simulink model "Copy_of_VTOLTiltrotor"  (R2024a)
settings: configuration reference "VTOLConfiguration" (kept outside this file)
undefined symbols (not defined in the file): airspeed, Battery, BCE12, BCE_Set_init, BMS_Controller_State, C, Cell10_P, Cell11_P, Cell12_P, Cell1_N, Cell1_P, Cell2_P, Cell3_P, Cell4_P, Cell5_P, Cell6_P, Cell7_P, Cell8_P, Cell9_P, Cell_Temperatures, Cell_Voltages, Charging_State, CityMission, control, controlParams, ControlSampleTime, CriticalTiltAngle, currentFactor, CV_Gain, ddx, ddy, ddz, Device_01, DiscIntNeverNeededParam, dx, dy, dz, Earth, env, F, F28379D_ADC_MaxCount, F28379D_ADC_Vmax, FixedWingMission, flightState, Foc_Ki_IxTcpu, Foc_Ki_S, Foc_Kp_I, Foc_Kp_S, fractalcoef, FSState, FWControlParams, HoverMission, I_cc, Ia_offset, Ib_offset, iniRoll, initPitch, iniYaw, IO334, IO334_DAC_Vmax ... (+55)
libraries: slrealtimeethercatlib x109, simulink x81, fl_lib x65, slpidlib x49, mcbcontrolslib x48, nesl_utility x43, speedgoatlib_hdlCoder_IO3xx x31, canmsglib x17, slrealtimeutilitieslib x13, mcbhdlplantlib x13, speedgoatlib_IO611 x12, dspstat3 x12
(part 8 of 20)

== system Copy_of_VTOLTiltrotor/Motor Control/Three-Phase PMSM Drive/PMSM and inverter with switching dynamics/PMSM_3P2L_Inverter_Plant_TBR ==
  PCIe_RC_or_TTL : Inport
  PCIe_PWM_Config : Inport  Port=2
  PCIe_PWM_Runtime : Inport  Port=3
  PCIe_PWM_Enable : Inport  Port=4
  PCIe_Protocol : Inport  Port=5
  PCIe_V_dc : Inport  Port=6
  PCIe_Fault : Inport  Port=7
  PCIe_LdTrq/Spd : Inport  Port=8
  PCIe_Motor_Config : Inport  Port=9
  PCIe_Motor_Connection : Inport  Port=10
  PCIe_QAE_Config : Inport  Port=11
  PCIe_Resolver_Config : Inport  Port=12
  PCIe_Iabc_DAC_gain : Inport  Port=13
  PCIe_Iabc_DAC_bias : Inport  Port=14
  PCIe_DAC_reset : Inport  Port=15
  HIL_PWM_{0..5} (6 alike) : Constant  Value=0  OutDataTypeStr=boolean
  PMSM_3P2L_Inverter_Plant1 : Subsystem  mask(Speedgoat IO334-325k Interface Block){module_id=1, slot=-1, ts=-1, dacGain_1=10.0V, dacActiv_1=off, dacGain_2=2.5V, dacActiv_2=on, dacGain_3=2.5V, dacActiv_3=on, dacGain_4=2.5V, dacActiv_4=on, dacGain_5=2.5V, dacActiv_5=on, dacGain_6=10.0V, dacActiv_6=off, dacGain_7=2.5V, dacActiv_7=on, dacGain_8=10.0V, dacActiv_8=off, dacGain_9=10.0V, dacActiv_9=off, dacGain_10=10.0V, dacActiv_10=off, dacGain_11=10.0V, dacActiv_11=off, dacGain_12=10.0V, dacActiv_12=off, dacGain_13=10.0V, dacActiv_13=off, dacGain_14=10.0V, dacActiv_14=off, dacGain_15=10.0V, dacActiv_15=off, dacGain_16=10.0V, dacActiv_16=off, PullRPort0=pull-up 3.3V, VioPort0=3.3V, PullRPort1=pull-up 3.3V, VioPort1=3.3V, PullRPort2=pull-up 3.3V, VioPort2=3.3V, PullRPort3=pull-up 3.3V, VioPort3=3.3V, PullRPort4=pull-up 3.3V, VioPort4=3.3V, PullRPort5=pull-up 3.3V, VioPort5=3.3V, PullRPort6=pull-up 3.3V, VioPort6=3.3V, fpga_sync_mode=on, reset_mode=on, reset_mode_stop=on, FpgaFreq=200}
      mask prompts: module_id "FPGA Module Identifier:"; slot "PCI slot (-1: autosearch):"; ts "Sample time:"; dacGain_1 "DAC Ch 01 Range"; dacActiv_1 "Activ"; dacGain_2 "DAC Ch 02 Range"; dacActiv_2 "Activ"; dacGain_3 "DAC Ch 03 Range"; dacActiv_3 "Activ"; dacGain_4 "DAC Ch 04 Range"; dacActiv_4 "Activ"; dacGain_5 "DAC Ch 05 Range"; dacActiv_5 "Activ"; dacGain_6 "DAC Ch 06 Range"; dacActiv_6 "Activ"; dacGain_7 "DAC Ch 07 Range"; dacActiv_7 "Activ"; dacGain_8 "DAC Ch 08 Range"; dacActiv_8 "Activ"; dacGain_9 "DAC Ch 09 Range"; dacActiv_9 "Activ"; dacGain_10 "DAC Ch 10 Range"; dacActiv_10 "Activ"; dacGain_11 "DAC Ch 11 Range"; dacActiv_11 "Activ"; dacGain_12 "DAC Ch 12 Range"; dacActiv_12 "Activ"; dacGain_13 "DAC Ch 13 Range"; dacActiv_13 "Activ"; dacGain_14 "DAC Ch 14 Range"; dacActiv_14 "Activ"; dacGain_15 "DAC Ch 15 Range"; dacActiv_15 "Activ"; dacGain_16 "DAC Ch 16 Range"; dacActiv_16 "Activ"; PullRPort0 "pull resistor"; VioPort0 "I/O voltage"; PullRPort1 "pull resistor"; VioPort1 "I/O voltage"; PullRPort2 "pull resistor"; VioPort2 "I/O voltage"; PullRPort3 "pull resistor"; VioPort3 "I/O voltage"; PullRPort4 "pull resistor"; VioPort4 "I/O voltage"; PullRPort5 "pull resistor"; VioPort5 "I/O voltage"; PullRPort6 "pull resistor"; VioPort6 "I/O voltage"; fpga_sync_mode "Run FPGA only when target application runs"; reset_mode "Reset FPGA states on start"; reset_mode_stop "Reset FPGA states on stop"; FpgaFreq "FPGA Frequency [MHz]"
      mask help: Simulink Real-Time Interface Block for Speedgoat IO334-325k.
      mask init:
      | hdlslrt.backend.mfpgaparameters;
      | if sg.hdlc.utils.compareMatlabVersion('~=', 'R2023b')
      | 	sg.hdlc.warning(['The interface model that you are attempting to use was generated ',...
      | 		'in MATLAB R2023b and may not be compatible with the version you are currently using. ',...
      | 		'Attempting to use this interface model in a different MATLAB release can lead to ',...
      | 		'application crashes or other unpredictable behavior. ',...
      | 		'In order to avoid this and ensure stability and correct functionality, ',...
      | 		'we highly recommend regenerating the model with your current MATLAB release.']);
      | end
      mask Help: eval('speedgoatdoc_hdlc')
      mask TypeOptions dacGain_1: AD5547 Setup/dacGain_1
      mask TypeOptions dacActiv_1: AD5547 Setup/dacActiv_1
      mask TypeOptions dacGain_2: AD5547 Setup/dacGain_2
      mask TypeOptions dacActiv_2: AD5547 Setup/dacActiv_2
      mask TypeOptions dacGain_3: AD5547 Setup/dacGain_3
      mask TypeOptions dacActiv_3: AD5547 Setup/dacActiv_3
      mask TypeOptions dacGain_4: AD5547 Setup/dacGain_4
      mask TypeOptions dacActiv_4: AD5547 Setup/dacActiv_4
      mask TypeOptions dacGain_5: AD5547 Setup/dacGain_5
      mask TypeOptions dacActiv_5: AD5547 Setup/dacActiv_5
      mask TypeOptions dacGain_6: AD5547 Setup/dacGain_6
      mask TypeOptions dacActiv_6: AD5547 Setup/dacActiv_6
      mask TypeOptions dacGain_7: AD5547 Setup/dacGain_7
      mask TypeOptions dacActiv_7: AD5547 Setup/dacActiv_7
      mask TypeOptions dacGain_8: AD5547 Setup/dacGain_8
      mask TypeOptions dacActiv_8: AD5547 Setup/dacActiv_8
      mask TypeOptions dacGain_9: AD5547 Setup/dacGain_9
      mask TypeOptions dacActiv_9: AD5547 Setup/dacActiv_9
      mask TypeOptions dacGain_10: AD5547 Setup/dacGain_10
      mask TypeOptions dacActiv_10: AD5547 Setup/dacActiv_10
      mask TypeOptions dacGain_11: AD5547 Setup/dacGain_11
      mask TypeOptions dacActiv_11: AD5547 Setup/dacActiv_11
      mask TypeOptions dacGain_12: AD5547 Setup/dacGain_12
      mask TypeOptions dacActiv_12: AD5547 Setup/dacActiv_12
      mask TypeOptions dacGain_13: AD5547 Setup/dacGain_13
      mask TypeOptions dacActiv_13: AD5547 Setup/dacActiv_13
      mask TypeOptions dacGain_14: AD5547 Setup/dacGain_14
      mask TypeOptions dacActiv_14: AD5547 Setup/dacActiv_14
      mask TypeOptions dacGain_15: AD5547 Setup/dacGain_15
      mask TypeOptions dacActiv_15: AD5547 Setup/dacActiv_15
      mask TypeOptions dacGain_16: AD5547 Setup/dacGain_16
      mask TypeOptions dacActiv_16: AD5547 Setup/dacActiv_16
      mask TypeOptions PullRPort0: Port Settings -2x 0x00590000/PullRPort0
      mask Callback PullRPort0: sg_fpga_HDLCoder_io3xx_2x_m(2);
      mask TypeOptions VioPort0: Port Settings -2x 0x00590000/VioPort0
      mask Callback VioPort0: sg_fpga_HDLCoder_io3xx_2x_m(2);
      mask TypeOptions PullRPort1: Port Settings -2x 0x00590000/PullRPort1
      mask Callback PullRPort1: sg_fpga_HDLCoder_io3xx_2x_m(2);
      mask TypeOptions VioPort1: Port Settings -2x 0x00590000/VioPort1
      mask Callback VioPort1: sg_fpga_HDLCoder_io3xx_2x_m(2);
      mask TypeOptions PullRPort2: Port Settings -2x 0x00590000/PullRPort2
      mask Callback PullRPort2: sg_fpga_HDLCoder_io3xx_2x_m(2);
      mask TypeOptions VioPort2: Port Settings -2x 0x00590000/VioPort2
      mask Callback VioPort2: sg_fpga_HDLCoder_io3xx_2x_m(2);
      mask TypeOptions PullRPort3: Port Settings -2x 0x00590000/PullRPort3
      mask Callback PullRPort3: sg_fpga_HDLCoder_io3xx_2x_m(2);
      mask TypeOptions VioPort3: Port Settings -2x 0x00590000/VioPort3
      mask Callback VioPort3: sg_fpga_HDLCoder_io3xx_2x_m(2);
      mask TypeOptions PullRPort4: Port Settings -2x 0x00590000/PullRPort4
      mask Callback PullRPort4: sg_fpga_HDLCoder_io3xx_2x_m(2);
      mask TypeOptions VioPort4: Port Settings -2x 0x00590000/VioPort4
      mask Callback VioPort4: sg_fpga_HDLCoder_io3xx_2x_m(2);
      mask TypeOptions PullRPort5: Port Settings -2x 0x00590000/PullRPort5
      mask Callback PullRPort5: sg_fpga_HDLCoder_io3xx_2x_m(2);
      mask TypeOptions VioPort5: Port Settings -2x 0x00590000/VioPort5
      mask Callback VioPort5: sg_fpga_HDLCoder_io3xx_2x_m(2);
      mask TypeOptions PullRPort6: Port Settings -2x 0x00590000/PullRPort6
      mask Callback PullRPort6: sg_fpga_HDLCoder_io3xx_2x_m(2);
      mask TypeOptions VioPort6: Port Settings -2x 0x00590000/VioPort6
      mask Callback VioPort6: sg_fpga_HDLCoder_io3xx_2x_m(2);
      mask TypeOptions fpga_sync_mode: IO3xx Setup/fpga_sync_mode
      mask TypeOptions reset_mode: IO3xx Setup/reset_mode
      mask TypeOptions reset_mode_stop: IO3xx Setup/reset_mode_stop
      mask DialogControl DAC Prompt: DAC
      mask DialogControl dacGrp_1 Prompt: Ch 01 to 08
      mask DialogControl dacGrp_2 Prompt: Ch 09 to 16
      mask DialogControl IO33421 Prompt: IO334-21
      mask DialogControl port1 Prompt: Port 1
      mask DialogControl port2 Prompt: Port 2
      mask DialogControl port3 Prompt: Port 3
      mask DialogControl port4 Prompt: Port 4
      mask DialogControl port5 Prompt: Port 5
      mask DialogControl port6 Prompt: Port 6
      mask DialogControl port7 Prompt: Port 7
      mask Display:
      | SetupBlkPath = sghdlc.model.findSystem(gcb, 'LookUnderMasks', 'all', 'FollowLinks', 'on', 'regexp', 'on', 'Name', 'IO3(\d|x){2}\s+Setup' );
      | SetupBlkPath = SetupBlkPath{1};
      | TS = get_param(SetupBlkPath,'timestamp_mcs');
      | disp(sprintf('Speedgoat IO334-325k\nFPGA I/O Module\n\nTimestamp\n%s\n\nReference Design\nVersion 1.0\n\nMATLAB R2023b\n\nPCIe Link Width: X4\nTiming Severity: error\nRear Plugin: -21\nAurora Mode: None\nAurora Crc: true\nAurora Byteswap: true\nVerifier: off\nVerifier: JTAG\n', TS))
  Terminator{,1..10} (11 alike) : Terminator
  PCIe_Ia : Outport
  PCIe_Ib : Outport  Port=2
  PCIe_Ic : Outport  Port=3
  PCIe_Idc : Outport  Port=4
  PCIe_Motor_Spd : Outport  Port=5
  PCIe_Motor_Angle : Outport  Port=6
  PCIe_Motor_ElecAngle : Outport  Port=7
  PCIe_Motor_Trq : Outport  Port=8
  PCIe_Rsvl_excitation_pos : Outport  Port=9
  PCIe_Rsvl_excitation_neg : Outport  Port=10
  PCIe_Rsvl_sin_neg : Outport  Port=11
  PCIe_Rsvl_cos_neg : Outport  Port=12
  PCIe_Resolver_Out : Outport  Port=13
  wires:
  PCIe_RC_or_TTL/1 -> PMSM_3P2L_Inverter_Plant1/1(PCIe_RC_or_TTL)
  PCIe_PWM_Config/1 -> PMSM_3P2L_Inverter_Plant1/2(PCIe_PWM_Config)
  PCIe_PWM_Runtime/1 -> PMSM_3P2L_Inverter_Plant1/3(PCIe_PWM_Runtime)
  PCIe_PWM_Enable/1 -> PMSM_3P2L_Inverter_Plant1/4(PCIe_PWM_Enable)
  PCIe_Protocol/1 -> PMSM_3P2L_Inverter_Plant1/5(PCIe_Protocol)
  PCIe_V_dc/1 -> PMSM_3P2L_Inverter_Plant1/12(PCIe_V_dc)
  PCIe_Fault/1 -> PMSM_3P2L_Inverter_Plant1/13(PCIe_Fault)
  PCIe_LdTrq/Spd/1 -> PMSM_3P2L_Inverter_Plant1/14(PCIe_LdTrq/Spd)
  PCIe_Motor_Config/1 -> PMSM_3P2L_Inverter_Plant1/15(PCIe_Motor_Config)
  PCIe_Motor_Connection/1 -> PMSM_3P2L_Inverter_Plant1/16(PCIe_Motor_Connection)
  PCIe_QAE_Config/1 -> PMSM_3P2L_Inverter_Plant1/17(PCIe_QAE_Config)
  PCIe_Resolver_Config/1 -> PMSM_3P2L_Inverter_Plant1/18(PCIe_Resolver_Config)
  PCIe_DAC_reset/1 -> PMSM_3P2L_Inverter_Plant1/21(PCIe_DAC_reset)
  PCIe_Iabc_DAC_bias/1 -> PMSM_3P2L_Inverter_Plant1/20(PCIe_Iabc_DAC_bias)
  PCIe_Iabc_DAC_gain/1 -> PMSM_3P2L_Inverter_Plant1/19(PCIe_Iabc_DAC_gain)
  PMSM_3P2L_Inverter_Plant1/1(PCIe_Ia) -> PCIe_Ia/1
  PMSM_3P2L_Inverter_Plant1/3(PCIe_Ic) -> PCIe_Ic/1
  PMSM_3P2L_Inverter_Plant1/2(PCIe_Ib) -> PCIe_Ib/1
  PMSM_3P2L_Inverter_Plant1/7(PCIe_Idc) -> PCIe_Idc/1
  PMSM_3P2L_Inverter_Plant1/8(PCIe_Motor_Spd) -> PCIe_Motor_Spd/1
  PMSM_3P2L_Inverter_Plant1/9(PCIe_Motor_Angle) -> PCIe_Motor_Angle/1
  PMSM_3P2L_Inverter_Plant1/10(PCIe_Motor_ElecAngle) -> PCIe_Motor_ElecAngle/1
  PMSM_3P2L_Inverter_Plant1/11(PCIe_Motor_Trq) -> PCIe_Motor_Trq/1
  PMSM_3P2L_Inverter_Plant1/15(PCIe_Rsvl_excitation_pos) -> PCIe_Rsvl_excitation_pos/1
  PMSM_3P2L_Inverter_Plant1/16(PCIe_Rsvl_excitation_neg) -> PCIe_Rsvl_excitation_neg/1
  PMSM_3P2L_Inverter_Plant1/17(AO_5_Rsvl_sin_pos) -> Terminator10/1  "F28379D_A5"
  PMSM_3P2L_Inverter_Plant1/18(PCIe_Rsvl_sin_neg) -> PCIe_Rsvl_sin_neg/1
  PMSM_3P2L_Inverter_Plant1/20(PCIe_Rsvl_cos_neg) -> PCIe_Rsvl_cos_neg/1
  PMSM_3P2L_Inverter_Plant1/21(PCIe_Resolver_Out) -> PCIe_Resolver_Out/1
  PMSM_3P2L_Inverter_Plant1/22(TTL_32_Protocol) -> Terminator/1  "GPIO40"
  PMSM_3P2L_Inverter_Plant1/23(TTL_24_AO_trigger_1_8) -> Terminator1/1
  PMSM_3P2L_Inverter_Plant1/24(1_8_Null_AO_trigger) -> Terminator2/1
  PMSM_3P2L_Inverter_Plant1/19(AO_7_Rsvl_cos_pos) -> Terminator3/1  "F28379D_C5"
  PMSM_3P2L_Inverter_Plant1/14("TTL_50_QEP_A_I   ") -> Terminator6/1
  PMSM_3P2L_Inverter_Plant1/12(TTL_48_QEP_A_A) -> Terminator4/1
  PMSM_3P2L_Inverter_Plant1/13(TTL_49_QEP_A_B) -> Terminator5/1
  PMSM_3P2L_Inverter_Plant1/6(AO_4_Ic) -> Terminator9/1  "F28379D_C4"
  PMSM_3P2L_Inverter_Plant1/4(AO_2_Ia) -> Terminator7/1  "F28379D_A4"
  PMSM_3P2L_Inverter_Plant1/5(AO_3_Ib) -> Terminator8/1  "F28379D_B4"
  HIL_PWM_0/1 -> PMSM_3P2L_Inverter_Plant1/6(PWM1A TTL_0)
  HIL_PWM_1/1 -> PMSM_3P2L_Inverter_Plant1/7(PWM1B TTL_1)
  HIL_PWM_2/1 -> PMSM_3P2L_Inverter_Plant1/8(PWM2A TTL_2)
  HIL_PWM_3/1 -> PMSM_3P2L_Inverter_Plant1/9(PWM2B TTL_3)
  HIL_PWM_4/1 -> PMSM_3P2L_Inverter_Plant1/10(PWM3A TTL_4)
  HIL_PWM_5/1 -> PMSM_3P2L_Inverter_Plant1/11(PWM3B TTL_5)

== system Copy_of_VTOLTiltrotor/Motor Control/Three-Phase PMSM Drive1/PMSM and average inverter/Encoder Simulation ==
  Theta_m : Inport
  Add1 : Sum  RndMeth=Simplest
  Data Type Conversion7 : DataTypeConversion  OutDataTypeStr=uint16  RndMeth=Simplest  SaturateOnIntegerOverflow=off
  "Get_PU " : Subsystem
  IndexOffset in PU : Constant  Value=0  OutDataTypeStr=single  SampleTime=-1
  Wrap : Subsystem
  pmsm.QEPSlits*4 : Gain  Gain=Maxon_Mile_Nslits*4  OutDataTypeStr=uint16  RndMeth=Simplest
  QEP_Position_Count : Outport
  wires:
  Add1/1 -> Wrap/1(in)
  Theta_m/1 -> "Get_PU "/1(rad)
  pmsm.QEPSlits*4/1 -> Data Type Conversion7/1  "Theta_e"
  Wrap/1(out) -> pmsm.QEPSlits*4/1  "theta_m(ideal)"
  IndexOffset in PU/1 -> Add1/2
  "Get_PU "/1(PU) -> Add1/1
  Data Type Conversion7/1 -> QEP_Position_Count/1

== system Copy_of_VTOLTiltrotor/Motor Control/Three-Phase PMSM Drive1/PMSM and average inverter/Ideal Inverter ==
  V_DC : Inport
  Duty Cycle abc : Inport  Port=2
  Data Type Conversion : DataTypeConversion  OutDataTypeStr=single  SaturateOnIntegerOverflow=off  RndMeth=Floor
  Demux : Demux  Outputs=3
  Mux : Mux  Inputs=3
  Product : Product
  Product1 : Product
  Product2 : Product
  Vabc : Outport
  wires:
  V_DC/1 -> Product2/1, Product1/1, Product/1
  Demux/1 -> Product/2
  Duty Cycle abc/1 -> Data Type Conversion/1
  Mux/1 -> Vabc/1
  Data Type Conversion/1 -> Demux/1
  Demux/2 -> Product1/2
  Demux/3 -> Product2/2
  Product/1 -> Mux/1
  Product1/1 -> Mux/2
  Product2/1 -> Mux/3

== system Copy_of_VTOLTiltrotor/Motor Control/Three-Phase PMSM Drive1/PMSM and average inverter/PMSM ==
  Config : Inport
  PhaseVolt abc : Inport  Port=2
  LdTrq / Spd : Inport  Port=3
  Constant : Constant  Value=0  OutDataTypeStr=boolean
  PMSM HDL : mcbhdlplantlib/PMSM HDL  VariantControl=pmsmVariant==pmsmEnum.TorqueInput  Ts=-1
      settings: LibrarySourceBlock=mcbhdllib/Electrical Systems/Motors/PMSM HDL
  Info : Outport
  PhaseCurr : Outport  Port=2
  Torque : Outport  Port=3
  RotorMechSpd : Outport  Port=4
  RotorElecAngle : Outport  Port=5
  wires:
  PMSM HDL/5 -> RotorElecAngle/1
  Config/1 -> PMSM HDL/1
  PMSM HDL/4 -> RotorMechSpd/1
  PMSM HDL/3 -> Torque/1
  PMSM HDL/2 -> PhaseCurr/1
  LdTrq / Spd/1 -> PMSM HDL/3
  PhaseVolt abc/1 -> PMSM HDL/2
  PMSM HDL/1 -> Info/1
  Constant/1 -> PMSM HDL/4

== system Copy_of_VTOLTiltrotor/Motor Control/Three-Phase PMSM Drive1/PMSM and average inverter/Runtime to DC ==
  PWM_Runtime : Inport
  Demux : Demux  Outputs=15
  Mux : Mux  Inputs=3
  To Dc A1 : Subsystem
  To Dc A2 : Subsystem
  To Dc A3 : Subsystem
  Duty Cycle abc : Outport
  wires:
  PWM_Runtime/1 -> Demux/1  "PCIe_PWM_Runtime"
  Demux/2 -> To Dc A1/1(A_on)
  Demux/3 -> To Dc A1/2(A_off)
  Demux/7 -> To Dc A2/1(A_on)
  Demux/8 -> To Dc A2/2(A_off)
  Demux/12 -> To Dc A3/1(A_on)
  Demux/13 -> To Dc A3/2(A_off)
  To Dc A1/1(Dc) -> Mux/1
  To Dc A2/1(Dc) -> Mux/2
  To Dc A3/1(Dc) -> Mux/3
  Mux/1 -> Duty Cycle abc/1

== system Copy_of_VTOLTiltrotor/Motor Control/Three-Phase PMSM Drive2/PMSM and average inverter/Encoder Simulation ==
  Theta_m : Inport
  Add1 : Sum  RndMeth=Simplest
  Data Type Conversion7 : DataTypeConversion  OutDataTypeStr=uint16  RndMeth=Simplest  SaturateOnIntegerOverflow=off
  "Get_PU " : Subsystem
  IndexOffset in PU : Constant  Value=0  OutDataTypeStr=single  SampleTime=-1
  Wrap : Subsystem
  pmsm.QEPSlits*4 : Gain  Gain=Maxon_Mile_Nslits*4  OutDataTypeStr=uint16  RndMeth=Simplest
  QEP_Position_Count : Outport
  wires:
  Add1/1 -> Wrap/1(in)
  Theta_m/1 -> "Get_PU "/1(rad)
  pmsm.QEPSlits*4/1 -> Data Type Conversion7/1  "Theta_e"
  Wrap/1(out) -> pmsm.QEPSlits*4/1  "theta_m(ideal)"
  IndexOffset in PU/1 -> Add1/2
  "Get_PU "/1(PU) -> Add1/1
  Data Type Conversion7/1 -> QEP_Position_Count/1

== system Copy_of_VTOLTiltrotor/Motor Control/Three-Phase PMSM Drive2/PMSM and average inverter/Ideal Inverter ==
  V_DC : Inport
  Duty Cycle abc : Inport  Port=2
  Data Type Conversion : DataTypeConversion  OutDataTypeStr=single  SaturateOnIntegerOverflow=off  RndMeth=Floor
  Demux : Demux  Outputs=3
  Mux : Mux  Inputs=3
  Product : Product
  Product1 : Product
  Product2 : Product
  Vabc : Outport
  wires:
  V_DC/1 -> Product2/1, Product1/1, Product/1
  Demux/1 -> Product/2
  Duty Cycle abc/1 -> Data Type Conversion/1
  Mux/1 -> Vabc/1
  Data Type Conversion/1 -> Demux/1
  Demux/2 -> Product1/2
  Demux/3 -> Product2/2
  Product/1 -> Mux/1
  Product1/1 -> Mux/2
  Product2/1 -> Mux/3

== system Copy_of_VTOLTiltrotor/Motor Control/Three-Phase PMSM Drive2/PMSM and average inverter/PMSM ==
  Config : Inport
  PhaseVolt abc : Inport  Port=2
  LdTrq / Spd : Inport  Port=3
  Constant : Constant  Value=0  OutDataTypeStr=boolean
  PMSM HDL : mcbhdlplantlib/PMSM HDL  VariantControl=pmsmVariant==pmsmEnum.TorqueInput  Ts=-1
      settings: LibrarySourceBlock=mcbhdllib/Electrical Systems/Motors/PMSM HDL
  Info : Outport
  PhaseCurr : Outport  Port=2
  Torque : Outport  Port=3
  RotorMechSpd : Outport  Port=4
  RotorElecAngle : Outport  Port=5
  wires:
  PMSM HDL/5 -> RotorElecAngle/1
  Config/1 -> PMSM HDL/1
  PMSM HDL/4 -> RotorMechSpd/1
  PMSM HDL/3 -> Torque/1
  PMSM HDL/2 -> PhaseCurr/1
  LdTrq / Spd/1 -> PMSM HDL/3
  PhaseVolt abc/1 -> PMSM HDL/2
  PMSM HDL/1 -> Info/1
  Constant/1 -> PMSM HDL/4

== system Copy_of_VTOLTiltrotor/Motor Control/Three-Phase PMSM Drive2/PMSM and average inverter/Runtime to DC ==
  PWM_Runtime : Inport
  Demux : Demux  Outputs=15
  Mux : Mux  Inputs=3
  To Dc A1 : Subsystem
  To Dc A2 : Subsystem
  To Dc A3 : Subsystem
  Duty Cycle abc : Outport
  wires:
  PWM_Runtime/1 -> Demux/1  "PCIe_PWM_Runtime"
  Demux/2 -> To Dc A1/1(A_on)
  Demux/3 -> To Dc A1/2(A_off)
  Demux/7 -> To Dc A2/1(A_on)
  Demux/8 -> To Dc A2/2(A_off)
  Demux/12 -> To Dc A3/1(A_on)
  Demux/13 -> To Dc A3/2(A_off)
  To Dc A1/1(Dc) -> Mux/1
  To Dc A2/1(Dc) -> Mux/2
  To Dc A3/1(Dc) -> Mux/3
  Mux/1 -> Duty Cycle abc/1

== system Copy_of_VTOLTiltrotor/Motor Control/Three-Phase PMSM Drive3/PMSM and average inverter/Encoder Simulation ==
  Theta_m : Inport
  Add1 : Sum  RndMeth=Simplest
  Data Type Conversion7 : DataTypeConversion  OutDataTypeStr=uint16  RndMeth=Simplest  SaturateOnIntegerOverflow=off
  "Get_PU " : Subsystem
  IndexOffset in PU : Constant  Value=0  OutDataTypeStr=single  SampleTime=-1
  Wrap : Subsystem
  pmsm.QEPSlits*4 : Gain  Gain=Maxon_Mile_Nslits*4  OutDataTypeStr=uint16  RndMeth=Simplest
  QEP_Position_Count : Outport
  wires:
  Add1/1 -> Wrap/1(in)
  Theta_m/1 -> "Get_PU "/1(rad)
  pmsm.QEPSlits*4/1 -> Data Type Conversion7/1  "Theta_e"
  Wrap/1(out) -> pmsm.QEPSlits*4/1  "theta_m(ideal)"
  IndexOffset in PU/1 -> Add1/2
  "Get_PU "/1(PU) -> Add1/1
  Data Type Conversion7/1 -> QEP_Position_Count/1

== system Copy_of_VTOLTiltrotor/Motor Control/Three-Phase PMSM Drive3/PMSM and average inverter/Ideal Inverter ==
  V_DC : Inport
  Duty Cycle abc : Inport  Port=2
  Data Type Conversion : DataTypeConversion  OutDataTypeStr=single  SaturateOnIntegerOverflow=off  RndMeth=Floor
  Demux : Demux  Outputs=3
  Mux : Mux  Inputs=3
  Product : Product
  Product1 : Product
  Product2 : Product
  Vabc : Outport
  wires:
  V_DC/1 -> Product2/1, Product1/1, Product/1
  Demux/1 -> Product/2
  Duty Cycle abc/1 -> Data Type Conversion/1
  Mux/1 -> Vabc/1
  Data Type Conversion/1 -> Demux/1
  Demux/2 -> Product1/2
  Demux/3 -> Product2/2
  Product/1 -> Mux/1
  Product1/1 -> Mux/2
  Product2/1 -> Mux/3

== system Copy_of_VTOLTiltrotor/Motor Control/Three-Phase PMSM Drive3/PMSM and average inverter/PMSM ==
  Config : Inport
  PhaseVolt abc : Inport  Port=2
  LdTrq / Spd : Inport  Port=3
  Constant : Constant  Value=0  OutDataTypeStr=boolean
  PMSM HDL : mcbhdlplantlib/PMSM HDL  VariantControl=pmsmVariant==pmsmEnum.TorqueInput  Ts=-1
      settings: LibrarySourceBlock=mcbhdllib/Electrical Systems/Motors/PMSM HDL
  Info : Outport
  PhaseCurr : Outport  Port=2
  Torque : Outport  Port=3
  RotorMechSpd : Outport  Port=4
  RotorElecAngle : Outport  Port=5
  wires:
  PMSM HDL/5 -> RotorElecAngle/1
  Config/1 -> PMSM HDL/1
  PMSM HDL/4 -> RotorMechSpd/1
  PMSM HDL/3 -> Torque/1
  PMSM HDL/2 -> PhaseCurr/1
  LdTrq / Spd/1 -> PMSM HDL/3
  PhaseVolt abc/1 -> PMSM HDL/2
  PMSM HDL/1 -> Info/1
  Constant/1 -> PMSM HDL/4

== system Copy_of_VTOLTiltrotor/Motor Control/Three-Phase PMSM Drive3/PMSM and average inverter/Runtime to DC ==
  PWM_Runtime : Inport
  Demux : Demux  Outputs=15
  Mux : Mux  Inputs=3
  To Dc A1 : Subsystem
  To Dc A2 : Subsystem
  To Dc A3 : Subsystem
  Duty Cycle abc : Outport
  wires:
  PWM_Runtime/1 -> Demux/1  "PCIe_PWM_Runtime"
  Demux/2 -> To Dc A1/1(A_on)
  Demux/3 -> To Dc A1/2(A_off)
  Demux/7 -> To Dc A2/1(A_on)
  Demux/8 -> To Dc A2/2(A_off)
  Demux/12 -> To Dc A3/1(A_on)
  Demux/13 -> To Dc A3/2(A_off)
  To Dc A1/1(Dc) -> Mux/1
  To Dc A2/1(Dc) -> Mux/2
  To Dc A3/1(Dc) -> Mux/3
  Mux/1 -> Duty Cycle abc/1

== system Copy_of_VTOLTiltrotor/Battery Management System/BMS/HIL/Controller/PLANT-Rx ==
  CAN Read : speedgoatlib_IO611/Legacy/CAN/CAN Read  id=1  sampleTime=-1  portSelection=2  messageType=CAN  BusOutput=off  protl=IO611  ptIdx=1  isFDMod=1
      settings: SourceProductName=IO611
  Data Type Conversion{,1..3} (4 alike) : DataTypeConversion  OutDataTypeStr=single  SaturateOnIntegerOverflow=off  RndMeth=Floor
  Messages : Subsystem
  While Iterator : WhileIterator  MaxIters=-1  WhileBlockType=do-while
  BMS_Faults : Outport
  Charging_State : Outport  Port=2
  BMS_State : Outport  Port=3
  SOC : Outport  Port=4
  Discharge_Current_Limit : Outport  Port=5
  Charge_Current_Limit : Outport  Port=6
  Charge_Current_Req : Outport  Port=7
  wires:
  CAN Read/2 -> Messages/4(ID_0x502), Messages/3(ID_0x501), Messages/2(ID_0x202), Messages/1(ID_0x201)
  CAN Read/1 -> While Iterator/1
  Messages/1(Discharge_Current_Limit) -> Data Type Conversion/1
  Messages/7(Charging_State) -> Charging_State/1
  Messages/2(Charge_Current_Limit) -> Data Type Conversion1/1
  Messages/3(Charge_Current_Req) -> Data Type Conversion2/1
  Messages/4(SOC) -> Data Type Conversion3/1
  Messages/6(BMS_State) -> BMS_State/1
  Data Type Conversion/1 -> Discharge_Current_Limit/1
  Data Type Conversion1/1 -> Charge_Current_Limit/1
  Data Type Conversion2/1 -> Charge_Current_Req/1
  Data Type Conversion3/1 -> SOC/1
  Messages/5(BMS_Faults) -> BMS_Faults/1

== system Copy_of_VTOLTiltrotor/Battery Management System/BMS/HIL/Controller/PLANT-Tx ==
  to_Controller : Inport
  to_Controller_SRE : Inport  Port=2
  12-Cell : Subsystem  VariantControl=Ns_Module == 12
  wires:
  to_Controller/1 -> 12-Cell/1(to_Controller)
  to_Controller_SRE/1 -> 12-Cell/2(to_Controller_SRE)

== system Copy_of_VTOLTiltrotor/Battery Management System/BMS/MIL/Cell Monitoring Unit/Balancing_Circuit ==
  Bal_Cmd_Controller : Inport
  12-Cell : Subsystem  VariantControl=Ns_Module == 12
  Cells : PMIOPort  Side=Left
  Balancing_Currents : Outport
  wires:
  Bal_Cmd_Controller/1 -> 12-Cell/1(Bal_Cmd_Controller)
  12-Cell/1(Balancing_Currents) -> Balancing_Currents/1
  connections:
  Cells/RConn1 -- 12-Cell/LConn1

== system Copy_of_VTOLTiltrotor/Battery Management System/BMS/MIL/Controller/BMS State Machine ==
  Discharge_Current_Limit : Inport
  Charge_Current_Limit : Inport  Port=2
  State_Request : Inport  Port=3  OutDataTypeStr=Enum: SRE
  Sensor_Values : Inport  Port=4
  Fault_Reset_Enable : Inport  Port=5
  Bus Selector : BusSelector  OutputSignals=Cell_Voltages,Pack_Voltage,Cell_Temperatures,Pack_Current
  Data Type Conversion : DataTypeConversion  OutDataTypeStr=boolean  SaturateOnIntegerOverflow=off  RndMeth=Floor
  State_Machine : Stateflow chart  TreatAsAtomicUnit=on  VariantControl=(default)
  Charge_Current_Req : Outport  OutMin=-100  OutMax=100  OutDataTypeStr=single  VectorParamsAs1DForOutWhenUnconnected=off
  Faults : Outport  Port=2  OutDataTypeStr=Bus: Faults  VectorParamsAs1DForOutWhenUnconnected=off  BusOutputAsStruct=on
  Charging_State : Outport  Port=3
  BMS_State : Outport  Port=4  OutDataTypeStr=Enum: BMS_Controller_State  VectorParamsAs1DForOutWhenUnconnected=off
  wires:
  State_Machine/2(Fault_out) -> Faults/1  "Faults"
  Bus Selector/1 -> State_Machine/4(Cell_Voltages)  "<Cell_Voltages>"
  State_Machine/1(ChargeCurrentReq) -> Charge_Current_Req/1  "Charge_Current_Req"
  State_Request/1 -> State_Machine/3(State_Request)
  Discharge_Current_Limit/1 -> State_Machine/1(DischargeCurrentLimit)
  Charge_Current_Limit/1 -> State_Machine/2(ChargeCurrentLimit)
  Bus Selector/3 -> State_Machine/6(Cell_Temperatures)  "<Cell_Temperatures>"
  Bus Selector/2 -> State_Machine/5(Pack_Voltage)  "<Pack_Voltage>"
  Bus Selector/4 -> State_Machine/7(Pack_Current)  "<Pack_Current>"
  Sensor_Values/1 -> Bus Selector/1
  Fault_Reset_Enable/1 -> Data Type Conversion/1
  Data Type Conversion/1 -> State_Machine/8(Fault_Reset_Enable)
  State_Machine/3(ChargeModeReq) -> Charging_State/1  "Charging_State"
  State_Machine/4(BMS_State) -> BMS_State/1  "BMS_State"

== system Copy_of_VTOLTiltrotor/Battery Management System/BMS/MIL/Controller/Balancing Logic ==
  BMS_State : Inport  OutDataTypeStr=Enum: BMS_Controller_State  PortDimensions=1
  Sensor_Values : Inport  Port=2
  Balancing : Stateflow chart  TreatAsAtomicUnit=on  VariantControl=(default)
  Bus Selector1 : BusSelector  OutputSignals=Cell_Voltages
  Bal_Cmd : Outport  OutDataTypeStr=boolean  PortDimensions=[1,NumModules*Ns_Module]  VectorParamsAs1DForOutWhenUnconnected=off
  wires:
  Balancing/1(Bal_Cmd) -> Bal_Cmd/1  "Bal_Cmd"
  Bus Selector1/1 -> Balancing/2(CellVoltages)  "<Cell_Voltages>"
  Sensor_Values/1 -> Bus Selector1/1
  BMS_State/1 -> Balancing/1(BMS_State)

== system Copy_of_VTOLTiltrotor/Battery Management System/BMS/MIL/Controller/Current Calculations ==
  BMS_Input : Inport
  Bus Selector : BusSelector  OutputSignals=Cell_Voltages,Cell_Temperatures
  Charge_Current_Limit_Calc : Subsystem
  Discharge_Current_Limit_Calc : Subsystem
  MinMax : MinMax
  MinMax1 : MinMax
  MinMax2 : MinMax  Function=max
  MinMax4 : MinMax  Function=max
  Discharge_Current_Limit : Outport
  Charge_Current_Limit : Outport  Port=2
  wires:
  MinMax/1 -> Discharge_Current_Limit_Calc/1(MinCellVolt)  "Min_Cell_Volt"
  MinMax4/1 -> Discharge_Current_Limit_Calc/3(MaxCellTemp), Charge_Current_Limit_Calc/3(MaxCellTemp)  "Max_Cell_Temp"
  MinMax1/1 -> Discharge_Current_Limit_Calc/2(MinCellTemp), Charge_Current_Limit_Calc/2(MinCellTemp)  "Min_Cell_Temp"
  MinMax2/1 -> Charge_Current_Limit_Calc/1(MaxCellVolt)  "Max_Cell_Volt"
  Discharge_Current_Limit_Calc/1(Discharge_Current_Limit) -> Discharge_Current_Limit/1  "Discharge_Current_Limit"
  Charge_Current_Limit_Calc/1(Charge_Current_Limit) -> Charge_Current_Limit/1  "Charge_Current_Limit"
  Bus Selector/1 -> MinMax/1, MinMax2/1  "<Cell_Voltages>"
  Bus Selector/2 -> MinMax4/1, MinMax1/1  "<Cell_Temperatures>"
  BMS_Input/1 -> Bus Selector/1

== system Copy_of_VTOLTiltrotor/Battery Management System/BMS/MIL/Controller/SOC Calculation ==
  BMS_State : Inport  OutDataTypeStr=Enum: BMS_Controller_State
  Sensor_Values : Inport  Port=2
  Bus Selector2 : BusSelector  OutputSignals=Pack_Current,Cell_Voltages,Cell_Temperatures
  Compare To Constant : simulink/Logic and Bit Operations/Compare To Constant  relop=~=  const=BMS_Controller_State.BMS_Fault  OutDataTypeStr=boolean
  Coulomb Counting : Subsystem  VariantControl=SocAlgo==1
  Gain : Gain  Gain=100
  Measurement Function : Subsystem  TreatAsAtomicUnit=on
  Mux : Mux  Inputs=3
  PackCurrent : Gain  Gain=-1
  State Transition Function : Subsystem  TreatAsAtomicUnit=on
  Temp : Selector  InputPortWidth=Ns_Module*NumModules  IndexOptions=Index vector (dialog)  Indices=1  OutputSizes=1
  UKF_EKF_1TC : Subsystem  VariantControl=CellType==1
  Volt : Selector  InputPortWidth=Ns_Module*NumModules  IndexOptions=Index vector (dialog)  Indices=1  OutputSizes=1
  SOC : Outport  OutDataTypeStr=single  VectorParamsAs1DForOutWhenUnconnected=off
  wires:
  Mux/1 -> Gain/1  "SOC"
  UKF_EKF_1TC/1(SOC_UKF) -> Mux/2  "SOC_UKF"
  BMS_State/1 -> Compare To Constant/1
  Coulomb Counting/1(SOC) -> Mux/1  "SOC_CC"
  Volt/1 -> UKF_EKF_1TC/1(Cell_Voltage)
  Temp/1 -> Coulomb Counting/2(Temp), State Transition Function/2(Temperature K), Measurement Function/2(Temperature (K))
  Compare To Constant/1 -> UKF_EKF_1TC/Enable
  UKF_EKF_1TC/2(SOC_EKF) -> Mux/3  "SOC_EKF"
  Bus Selector2/1 -> Coulomb Counting/1(Curr), PackCurrent/1  "<Pack_Current>"
  PackCurrent/1 -> State Transition Function/1(Current), Measurement Function/1(Current)  "PackCurrent"
  Bus Selector2/3 -> Temp/1  "<Cell_Temperatures>"
  Bus Selector2/2 -> Volt/1  "<Cell_Voltages>"
  Sensor_Values/1 -> Bus Selector2/1
  Gain/1 -> SOC/1

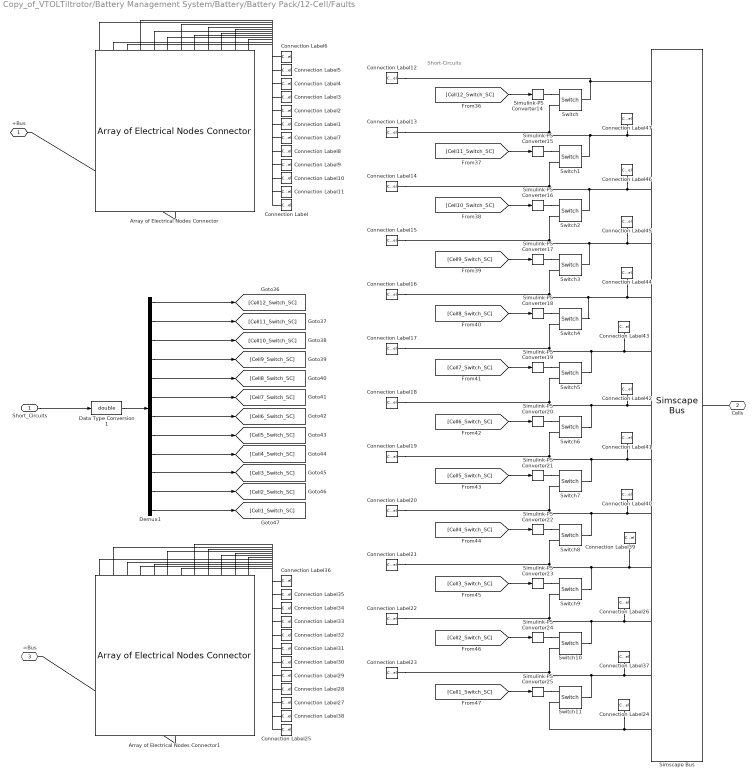
== system Copy_of_VTOLTiltrotor/Battery Management System/Battery/Battery Pack/12-Cell/Faults ==
  note: Short-Circuits
  Short_Circuits : Inport
  Array of Electrical Nodes Connector : batt_lib/Connectors/Array of Electrical Nodes Connector  numInputConnections=simscape.battery.enum.thermal.numArrayOfNodesConnections.twelve  inNode1NumElements=1  inNode2NumElements=1  inNode3NumElements=1  inNode4NumElements=1  inNode5NumElements=1  inNode6NumElements=1  inNode7NumElements=1  inNode8NumElements=1  inNode9NumElements=1  inNode10NumElements=1  inNode11NumElements=1  inNode12NumElements=1  inNode13NumElements=1  inNode14NumElements=1  inNode15NumElements=1  inNode16NumElements=1  inNode17NumElements=1  inNode18NumElements=1  inNode19NumElements=1  inNode20NumElements=1  inNode21NumElements=1  inNode22NumElements=1  inNode23NumElements=1  inNode24NumElements=1  inNode25NumElements=1  inNode26NumElements=1  inNode27NumElements=1  inNode28NumElements=1  inNode29NumElements=1  inNode30NumElements=1  inNode31NumElements=1  inNode32NumElements=1  inNode33NumElements=1  inNode34NumElements=1  inNode35NumElements=1  inNode36NumElements=1  inNode37NumElements=1  inNode38NumElements=1  inNode39NumElements=1  inNode40NumElements=1  inNode41NumElements=1  inNode42NumElements=1  inNode43NumElements=1  inNode44NumElements=1  inNode45NumElements=1  inNode46NumElements=1  inNode47NumElements=1  inNode48NumElements=1  inNode49NumElements=1  inNode50NumElements=1
      settings: InternalSimscapePortConfiguration="{\"Bottom\":[{\"id\":\"outConn\",\"label\":\"outConn\",\"type\":\"foundation.electrical.electrical\"}],\"Left\":[],\"Right\":[],\"Top\":[{\"id\":\"inConn1\",\"label\":\"inConn1\",\"type\":\"foundation.electrical.electrical\"},{\"id\":\"inConn2\",\"label\":\"inConn2\",\"type\":\"foundation.electrical.electrical\"},{\"id\":\"inConn3\",\"label\":\"inConn3\",\"type\":\"foundation.electrical.electrical\"},{\"id\":\"inConn4\",\"label\":\"inConn4\",\"type\":\"foundation.electrical.electrical\"},{\"id\":\"inConn5\",\"label\":\"inConn5\",\"type\":\"foundation.electrical.electrical\"},{\"id\":\"inConn6\",\"label\":\"inConn6\",\"type\":\"foundation.electrical.electrical\"},{\"id\":\"inConn7\",\"label\":\"inConn7\",\"type\":\"foundation.electrical.electrical\"},{\"id\":\"inConn8\",\"label\":\"inConn8\",\"type\":\"foundation.electrical.electrical\"},{\"id\":\"inConn9\",\"label\":\"inConn9\",\"type\":\"foundation.electrical.electrical\"},{\"id\":\"inConn10\",\"label\":\"inConn10\",\"type\":\"foundation.electrical.electrical\"},{\"id\":\"inConn11\",\"label\":\"inConn11\",\"type\":\"foundation.electrical.electrical\"},{\"id\":\"inConn12\",\"label\":\"inConn12\",\"type\":\"foundation.electrical.electrical\"}]}"
  Array of Electrical Nodes Connector1 : batt_lib/Connectors/Array of Electrical Nodes Connector  numInputConnections=simscape.battery.enum.thermal.numArrayOfNodesConnections.twelve  inNode1NumElements=1  inNode2NumElements=1  inNode3NumElements=1  inNode4NumElements=1  inNode5NumElements=1  inNode6NumElements=1  inNode7NumElements=1  inNode8NumElements=1  inNode9NumElements=1  inNode10NumElements=1  inNode11NumElements=1  inNode12NumElements=1  inNode13NumElements=1  inNode14NumElements=1  inNode15NumElements=1  inNode16NumElements=1  inNode17NumElements=1  inNode18NumElements=1  inNode19NumElements=1  inNode20NumElements=1  inNode21NumElements=1  inNode22NumElements=1  inNode23NumElements=1  inNode24NumElements=1  inNode25NumElements=1  inNode26NumElements=1  inNode27NumElements=1  inNode28NumElements=1  inNode29NumElements=1  inNode30NumElements=1  inNode31NumElements=1  inNode32NumElements=1  inNode33NumElements=1  inNode34NumElements=1  inNode35NumElements=1  inNode36NumElements=1  inNode37NumElements=1  inNode38NumElements=1  inNode39NumElements=1  inNode40NumElements=1  inNode41NumElements=1  inNode42NumElements=1  inNode43NumElements=1  inNode44NumElements=1  inNode45NumElements=1  inNode46NumElements=1  inNode47NumElements=1  inNode48NumElements=1  inNode49NumElements=1  inNode50NumElements=1
      settings: InternalSimscapePortConfiguration="{\"Bottom\":[{\"id\":\"outConn\",\"label\":\"outConn\",\"type\":\"foundation.electrical.electrical\"}],\"Left\":[],\"Right\":[],\"Top\":[{\"id\":\"inConn1\",\"label\":\"inConn1\",\"type\":\"foundation.electrical.electrical\"},{\"id\":\"inConn2\",\"label\":\"inConn2\",\"type\":\"foundation.electrical.electrical\"},{\"id\":\"inConn3\",\"label\":\"inConn3\",\"type\":\"foundation.electrical.electrical\"},{\"id\":\"inConn4\",\"label\":\"inConn4\",\"type\":\"foundation.electrical.electrical\"},{\"id\":\"inConn5\",\"label\":\"inConn5\",\"type\":\"foundation.electrical.electrical\"},{\"id\":\"inConn6\",\"label\":\"inConn6\",\"type\":\"foundation.electrical.electrical\"},{\"id\":\"inConn7\",\"label\":\"inConn7\",\"type\":\"foundation.electrical.electrical\"},{\"id\":\"inConn8\",\"label\":\"inConn8\",\"type\":\"foundation.electrical.electrical\"},{\"id\":\"inConn9\",\"label\":\"inConn9\",\"type\":\"foundation.electrical.electrical\"},{\"id\":\"inConn10\",\"label\":\"inConn10\",\"type\":\"foundation.electrical.electrical\"},{\"id\":\"inConn11\",\"label\":\"inConn11\",\"type\":\"foundation.electrical.electrical\"},{\"id\":\"inConn12\",\"label\":\"inConn12\",\"type\":\"foundation.electrical.electrical\"}]}"
  Connection Label : ConnectionLabel  Label=pos1
  Connection Label1 : ConnectionLabel  Label=pos7
  Connection Label10 : ConnectionLabel  Label=pos3
  Connection Label11 : ConnectionLabel  Label=pos2
  Connection Label12 : ConnectionLabel  Label=pos12
  Connection Label13 : ConnectionLabel  Label=pos11
  Connection Label14 : ConnectionLabel  Label=pos10
  Connection Label15 : ConnectionLabel  Label=pos9
  Connection Label16 : ConnectionLabel  Label=pos8
  Connection Label17 : ConnectionLabel  Label=pos7
  Connection Label18 : ConnectionLabel  Label=pos6
  Connection Label19 : ConnectionLabel  Label=pos5
  Connection Label2 : ConnectionLabel  Label=pos8
  Connection Label20 : ConnectionLabel  Label=pos4
  Connection Label21 : ConnectionLabel  Label=pos3
  Connection Label22 : ConnectionLabel  Label=pos2
  Connection Label23 : ConnectionLabel  Label=pos1
  Connection Label24 : ConnectionLabel  Label=neg1
  Connection Label25 : ConnectionLabel  Label=neg1
  Connection Label26 : ConnectionLabel  Label=neg3
  Connection Label27 : ConnectionLabel  Label=neg3
  Connection Label28 : ConnectionLabel  Label=neg4
  Connection Label29 : ConnectionLabel  Label=neg5
  Connection Label3 : ConnectionLabel  Label=pos9
  Connection Label30 : ConnectionLabel  Label=neg6
  Connection Label31 : ConnectionLabel  Label=neg7
  Connection Label32 : ConnectionLabel  Label=neg8
  Connection Label33 : ConnectionLabel  Label=neg9
  Connection Label34 : ConnectionLabel  Label=neg10
  Connection Label35 : ConnectionLabel  Label=neg11
  Connection Label36 : ConnectionLabel  Label=neg12
  Connection Label37 : ConnectionLabel  Label=neg2
  Connection Label38 : ConnectionLabel  Label=neg2
  Connection Label39 : ConnectionLabel  Label=neg4
  Connection Label4 : ConnectionLabel  Label=pos10
  Connection Label40 : ConnectionLabel  Label=neg5
  Connection Label41 : ConnectionLabel  Label=neg6
  Connection Label42 : ConnectionLabel  Label=neg7
  Connection Label43 : ConnectionLabel  Label=neg8
  Connection Label44 : ConnectionLabel  Label=neg9
  Connection Label45 : ConnectionLabel  Label=neg10
  Connection Label46 : ConnectionLabel  Label=neg11
  Connection Label47 : ConnectionLabel  Label=neg12
  Connection Label5 : ConnectionLabel  Label=pos11
  Connection Label6 : ConnectionLabel  Label=pos12
  Connection Label7 : ConnectionLabel  Label=pos6
  Connection Label8 : ConnectionLabel  Label=pos5
  Connection Label9 : ConnectionLabel  Label=pos4
  Data Type Conversion1 : DataTypeConversion  OutDataTypeStr=double  SaturateOnIntegerOverflow=off  RndMeth=Floor
  Demux1 : Demux  Outputs=12
  Simscape Bus : SimscapeBus  HierarchyStrings=Cell12_P;Cell11_P;Cell10_P;Cell9_P;Cell8_P;Cell7_P;Cell6_P;Cell5_P;Cell4_P;Cell3_P;Cell2_P;Cell1_P;Cell1_N
  Simulink-PS Converter{14..25} (12 alike) : nesl_utility/Simulink-PS Converter  PhysicalDomain=network_engine_domain  SubClassName=ps_input  LeftPortType=input  RightPortType=output  PseudoPeriodic=off  Frequencies=[]  NoiseDistribution=none  NoiseParameters=[]  Unit=1  AffineConversion=off  FilteringAndDerivatives=zero  SimscapeFilterOrder=1  InputFilterTimeConstant=0.001  UdotUserProvided=1
  Switch{,1..11} (12 alike) : fl_lib/Electrical/Electrical Elements/Switch  R_closed=0.01 Ohm  G_open=1e-8 1/Ohm  Threshold=0.5  i_specify=off  i_priority=None  i=0 A  i_nominal_specify=off  i_nominal_value=1  i_nominal_unit=A  v_specify=off  v_priority=None  v=0 V  v_nominal_specify=off  v_nominal_value=1  v_nominal_unit=V
  +Bus : PMIOPort  Side=Right
  Cells : PMIOPort  Port=2  Side=Right
  =Bus : PMIOPort  Port=3  Side=Right
  wires:
  [Cell2_Switch_SC] -> Simulink-PS Converter24/1
  [Cell3_Switch_SC] -> Simulink-PS Converter23/1
  Demux1/9 -> [Cell4_Switch_SC]
  Data Type Conversion1/1 -> Demux1/1
  Demux1/5 -> [Cell8_Switch_SC]
  Demux1/8 -> [Cell5_Switch_SC]
  [Cell1_Switch_SC] -> Simulink-PS Converter25/1
  [Cell12_Switch_SC] -> Simulink-PS Converter14/1
  [Cell11_Switch_SC] -> Simulink-PS Converter15/1
  Demux1/1 -> [Cell12_Switch_SC]
  Demux1/7 -> [Cell6_Switch_SC]
  [Cell4_Switch_SC] -> Simulink-PS Converter22/1
  Demux1/10 -> [Cell3_Switch_SC]
  Demux1/2 -> [Cell11_Switch_SC]
  [Cell8_Switch_SC] -> Simulink-PS Converter18/1
  [Cell5_Switch_SC] -> Simulink-PS Converter21/1
  Demux1/12 -> [Cell1_Switch_SC]
  [Cell10_Switch_SC] -> Simulink-PS Converter16/1
  [Cell9_Switch_SC] -> Simulink-PS Converter17/1
  Demux1/3 -> [Cell10_Switch_SC]
  Demux1/6 -> [Cell7_Switch_SC]
  [Cell6_Switch_SC] -> Simulink-PS Converter20/1
  [Cell7_Switch_SC] -> Simulink-PS Converter19/1
  Demux1/4 -> [Cell9_Switch_SC]
  Demux1/11 -> [Cell2_Switch_SC]
  Short_Circuits/1 -> Data Type Conversion1/1
  connections:
  Simulink-PS Converter17/RConn1 -- Switch3/RConn1
  Connection Label10/LConn1 -- Array of Electrical Nodes Connector/LConn10
  Switch3/LConn1 -- Connection Label45/LConn1 -- Simscape Bus/LConn4 -- Connection Label15/LConn1 -- Switch2/RConn2
  Switch6/LConn1 -- Connection Label42/LConn1 -- Simscape Bus/LConn7 -- Connection Label18/LConn1 -- Switch5/RConn2
  Connection Label31/LConn1 -- Array of Electrical Nodes Connector1/LConn6
  Switch7/LConn1 -- Connection Label41/LConn1 -- Simscape Bus/LConn8 -- Connection Label19/LConn1 -- Switch6/RConn2
  Switch2/LConn1 -- Connection Label46/LConn1 -- Simscape Bus/LConn3 -- Connection Label14/LConn1 -- Switch1/RConn2
  Connection Label28/LConn1 -- Array of Electrical Nodes Connector1/LConn9
  Connection Label29/LConn1 -- Array of Electrical Nodes Connector1/LConn8
  Simulink-PS Converter16/RConn1 -- Switch2/RConn1
  Simulink-PS Converter19/RConn1 -- Switch5/RConn1
  Switch10/LConn1 -- Connection Label26/LConn1 -- Simscape Bus/LConn11 -- Connection Label22/LConn1 -- Switch9/RConn2
  Simulink-PS Converter25/RConn1 -- Switch11/RConn1
  Connection Label27/LConn1 -- Array of Electrical Nodes Connector1/LConn10
  Connection Label25/LConn1 -- Array of Electrical Nodes Connector1/LConn12
  Switch11/LConn1 -- Connection Label37/LConn1 -- Simscape Bus/LConn12 -- Connection Label23/LConn1 -- Switch10/RConn2
  Connection Label39/LConn1 -- Simscape Bus/LConn10 -- Switch9/LConn1 -- Connection Label21/LConn1 -- Switch8/RConn2
  Connection Label36/LConn1 -- Array of Electrical Nodes Connector1/LConn1
  Connection Label34/LConn1 -- Array of Electrical Nodes Connector1/LConn3
  Connection Label35/LConn1 -- Array of Electrical Nodes Connector1/LConn2
  Simulink-PS Converter14/RConn1 -- Switch/RConn1
  Simscape Bus/LConn13 -- Connection Label24/LConn1 -- Switch11/RConn2
  Connection Label30/LConn1 -- Array of Electrical Nodes Connector1/LConn7
  Simulink-PS Converter18/RConn1 -- Switch4/RConn1
  Connection Label44/LConn1 -- Simscape Bus/LConn5 -- Switch4/LConn1 -- Connection Label16/LConn1 -- Switch3/RConn2
  Simulink-PS Converter24/RConn1 -- Switch10/RConn1
  Connection Label33/LConn1 -- Array of Electrical Nodes Connector1/LConn4
  Connection Label38/LConn1 -- Array of Electrical Nodes Connector1/LConn11
  Connection Label32/LConn1 -- Array of Electrical Nodes Connector1/LConn5
  Switch8/LConn1 -- Connection Label40/LConn1 -- Simscape Bus/LConn9 -- Connection Label20/LConn1 -- Switch7/RConn2
  Cells/RConn1 -- Simscape Bus/RConn1
  Simulink-PS Converter20/RConn1 -- Switch6/RConn1
  Simulink-PS Converter15/RConn1 -- Switch1/RConn1
  Simulink-PS Converter21/RConn1 -- Switch7/RConn1
  Simulink-PS Converter23/RConn1 -- Switch9/RConn1
  Simulink-PS Converter22/RConn1 -- Switch8/RConn1
  Connection Label11/LConn1 -- Array of Electrical Nodes Connector/LConn11
  Connection Label6/LConn1 -- Array of Electrical Nodes Connector/LConn1
  Connection Label7/LConn1 -- Array of Electrical Nodes Connector/LConn7
  Switch5/LConn1 -- Connection Label43/LConn1 -- Simscape Bus/LConn6 -- Connection Label17/LConn1 -- Switch4/RConn2
  Connection Label2/LConn1 -- Array of Electrical Nodes Connector/LConn5
  Simscape Bus/LConn1 -- Connection Label12/LConn1 -- Switch/LConn1
  Connection Label4/LConn1 -- Array of Electrical Nodes Connector/LConn3
  Connection Label8/LConn1 -- Array of Electrical Nodes Connector/LConn8
  Connection Label5/LConn1 -- Array of Electrical Nodes Connector/LConn2
  Connection Label3/LConn1 -- Array of Electrical Nodes Connector/LConn4
  Connection Label1/LConn1 -- Array of Electrical Nodes Connector/LConn6
  Connection Label/LConn1 -- Array of Electrical Nodes Connector/LConn12
  Connection Label9/LConn1 -- Array of Electrical Nodes Connector/LConn9
  Connection Label47/LConn1 -- Simscape Bus/LConn2 -- Switch1/LConn1 -- Connection Label13/LConn1 -- Switch/RConn2
  Array of Electrical Nodes Connector1/RConn1 -- =Bus/RConn1
  Array of Electrical Nodes Connector/RConn1 -- +Bus/RConn1
